simulink model "turbine"  (R2018b)
settings: Solver=ode1  StartTime=0.0  StopTime=100  FixedStep=0.1  RelTol=1e-3
PostLoadFcn:
  | , if any(exist('dsrtsu_mdlpostloadfcn', 'file') ~= 0), dsrtsu_mdlpostloadfcn('Execute', bdroot); end,
undefined symbols (not defined in the file): XXX
libraries: rtiethernetudplib x2
Description:
  | Standard RTI1401 template.
  | Supported MATLAB version:  R2018b.
settings Model: Tag=RTI1401  DSRTSU_INTERNAL_RTI_VER=530  DSRTSU_INTERNAL_RTI_TYPE=rti1401  RTICANMMDATA=struct('GeneralSetupData',struct('modelroot','C:\Users\akohlheb\working_files\OFF_RTS_PLC_API\dSpace','generalsettings',struct('filesettings',struct('destfolder',struct('Name','RTICANMM_FILES','Check',1),'buildfolder',struct('Name','.','Check',1),'AbsDestfolder',struct('Name','C:\Users\akohlheb\working_files\OFF_RTS_PLC_API\dSpace\RTICANMM_FILES'),'AbsBuildfolder',struct('Name','C:\Users\akohlheb\working_files\OFF_RTS_PLC_API\dSpace'))),'options',struct('addpaths',1,'rmpaths',1,'addtrcexclusion',logical(1),'cannavigator',struct('checkmonitoring',0),'show_usrtrc',0,'use_usrtrc',0),'advanced',struct('options',ones(1,100)),'MPSetup',{{}},'RTI',struct('Type','RTI1401','Ver','7.11','Date','02-Nov-2018'),'modelname','turbine','block','turbine'))  DSRTSU_INTERNAL_RTIFPGA=120  Creator=akohlheb  LastModifiedBy=akohlheb
settings OptimizationCC: BlockReduction=off  OptimizeBlockIOStorage=off  BufferReuse=off  GlobalBufferReuse=off  ExpressionFolding=off  LocalBlockOutputs=off  OptimizeDataStoreBuffers=off  BusAssignmentInplaceUpdate=off
settings DebuggingCC: LibraryContextMissingDiagnostic=none
settings HardwareCC: ProdBitPerPointer=32  ProdBitPerSizeT=32  ProdBitPerPtrDiffT=32  ProdLargestAtomicInteger=Integer  ProdEndianess=BigEndian  ProdWordSize=32  ProdHWDeviceType=Custom Processor->Custom  TargetIntDivRoundTo=Zero  TargetEndianess=BigEndian  TargetHWDeviceType=Custom Processor->Custom
settings SFSimCC: SimUseLocalCustomCode=off  MATLABDynamicMemAlloc=off
settings RTWCC: SystemTargetFile=rti1401.tlc  MakeCommand=make_rti  TemplateMakefile=rti1401.tmf  Description=dSPACE DS1401 Hardware Platform  RTWUseLocalCustomCode=off
settings CodeAppCC: StateflowObjectComments=on
settings STFCustomTargetCC: ParMdlRefBuildCompliant=on  SystemTargetFile=rti1401.tlc
settings GRTTargetCC: TargetLangStandard=C89/C90 (ANSI)  CompOptLevelCompliant=off  ConcurrentExecutionCompliant=off  CombineOutputUpdateFcns=off  MatFileLogging=off  CPPClassGenCompliant=off  UseToolchainInfoCompliant=off
settings ConfigComp: CovMetricSettings=dswe

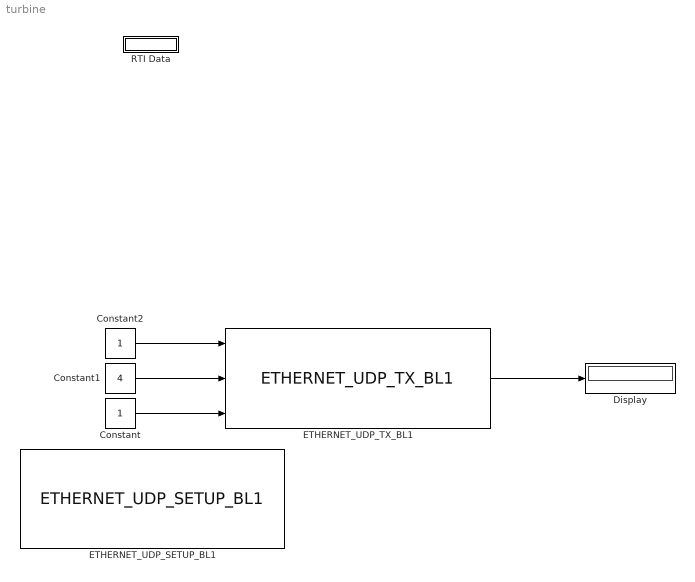
== system turbine ==
  Constant : Constant  OutDataTypeStr=boolean
  Constant1 : Constant  Value=4  OutDataTypeStr=int32
  Constant2 : Constant  OutDataTypeStr=uint32
  Display : Display
  ETHERNET_UDP_SETUP_BL1 : rtiethernetudplib/ETHERNET_UDP_SETUP_BL1  DSProperties=struct('RTI',struct('Version',uint32(1),'BlockType',struct('isSLSource',uint8(0),'isSLSink',uint8(0),'isHWSource',uint8(0),'isHWSink',uint8(0),'isSetup',uint8(0),'isInline',uint8(1),'isNonInline',uint8(1),'isInterrupt',uint8(0),'isChannelwise',uint8(0)),'IOBoardType','DSETHERNETUDP','UnitType','ETHUDP','Identifier','SETUP','DialogType','ML','BlockSet','RTIETHERNETUDP','SlaveProcessor','NONE'))  RTIBlockInterface=struct('OutputPortsActive',0,'OutputPortsWidth',int32(1),'DialogFcn','rtiethernetudpsetupgui','InitLevel',3,'BlockDisplay',{{['Ethernet UDP Setup\nInterface Name: rti_ethernet_interface_name\nBoard Type: ETH Type 1\nModule: 1\nLocal IP Address: XXX.XXX.XXX.XXX'],'center'}},'IconTransparency','on','BlockName',struct('Token',{{'ETHERNET_UDP_SETUP_BL1'}}))  RTIBlockParameters=struct('BoardType',{{1,'OFF',[]}},'ModuleNo',{{1,'ON',[1 16]}},'ChannelNo',{{1,'ON',[1 2]}},'InterfaceName',{{'rti_ethernet_interface_name','OFF',[]}},'LocalIpAddress',{{'XXX.XXX.XXX.XXX','OFF',[]}},'EnableSocket1',{{0,'OFF',[0 1]}},'LocalPortSocket1',{{5000,'OFF',[0 65535]}},'RemoteIpAddrSocket1',{{'XXX.XXX.XXX.XXX','OFF',[]}},'RemotePortSocket1',{{5000,'OFF',[0 65535]}},'EnableSocket2',{{0,'OFF',[0 1]}},'LocalPortSocket2',{{5001,'OFF',[0 65535]}},'RemoteIpAddrSocket2',{{'XXX.XXX.XXX.XXX','OFF',[]}},'RemotePortSocket2',{{5001,'OFF',[0 65535]}},'EnableSocket3',{{0,'OFF',[0 1]}},'LocalPortSocket3',{{5002,'OFF',[0 65535]}},'RemoteIpAddrSocket3',{{'XXX.XXX.XXX.XXX','OFF',[]}},'RemotePortSocket3',{{5002,'OFF',[0 65535]}},'EnableSocket4',{{0,'OFF',[0 1]}},'LocalPortSocket4',{{5003,'OFF',[0 65535]}},'RemoteIpAddrSocket4',{{'XXX.XXX.XXX.XXX','OFF',[]}},'RemotePortSocket4',{{5003,'OFF',[0 65535]}},'LocalIpAddrHex',{{0,'OFF',[]}},'RemoteIpAddrSocket1Hex',{{0,'OFF',[]}},'RemoteIpAddrSocket2Hex',{{0,'OFF',[]}},'RemoteIpAddrSocket3Hex',{{0,'OFF',[]}},'RemoteIpAddrSocket4Hex',{{0,'OFF',[]}})  RTISFcnParameters=struct('BoardType','double','ModuleNo','double','ChannelNo','double','InterfaceName','char','LocalIpAddress','char','EnableSocket1','double','LocalPortSocket1','double','RemoteIpAddrSocket1','char','RemotePortSocket1','double','EnableSocket2','double','LocalPortSocket2','double','RemoteIpAddrSocket2','char','RemotePortSocket2','double','EnableSocket3','double','LocalPortSocket3','double','RemoteIpAddrSocket3','char','RemotePortSocket3','double','EnableSocket4','double','LocalPortSocket4','double','RemoteIpAddrSocket4','char','RemotePortSocket4','double','LocalIpAddrHex','double','RemoteIpAddrSocket1Hex','double','RemoteIpAddrSocket2Hex','double','RemoteIpAddrSocket3Hex','double','RemoteIpAddrSocket4Hex','double')  RTIBlockParaDefault=struct('BoardType',1,'ModuleNo',1,'ChannelNo',1,'InterfaceName','rti_ethernet_interface_name','LocalIpAddress','XXX.XXX.XXX.XXX','EnableSocket1',0,'LocalPortSocket1',5000,'RemoteIpAddrSocket1','XXX.XXX.XXX.XXX','RemotePortSocket1',5000,'EnableSocket2',0,'LocalPortSocket2',5001,'RemoteIpAddrSocket2','XXX.XXX.XXX.XXX','RemotePortSocket2',5001,'EnableSocket3',0,'LocalPortSocket3',5002,'RemoteIpAddrSocket3','XXX.XXX.XXX.XXX','RemotePortSocket3',5002,'EnableSocket4',0,'LocalPortSocket4',5003,'RemoteIpAddrSocket4','XXX.XXX.XXX.XXX','RemotePortSocket4',5003,'LocalIpAddrHex',0,'RemoteIpAddrSocket1Hex',0,'RemoteIpAddrSocket2Hex',0,'RemoteIpAddrSocket3Hex',0,'RemoteIpAddrSocket4Hex',0)
      settings: SourceProductName=dSPACE RTI Ethernet (UDP) Blockset
  ETHERNET_UDP_TX_BL1 : rtiethernetudplib/ETHERNET_UDP_TX_BL1  InterfaceName=rti_ethernet_interface_name  BoardType=ETH Type 1  ModuleNo=1  ChannelNo=1  SocketNo=1  MaxMessageSize=4  SendTimeout=0.0005  LocalSocket=XXX.XXX.XXX.XXX:5000  RemoteSocket=XXX.XXX.XXX.XXX:5000  DSProperties=struct('RTI',struct('Version',uint32(2),'BlockType',struct('isSLSource',uint8(1),'isSLSink',uint8(1),'isHWSource',uint8(1),'isHWSink',uint8(1),'isSetup',uint8(0),'isInline',uint8(1),'isNonInline',uint8(1),'isInterrupt',uint8(0),'isChannelwise',uint8(1)),'IOBoardType','DSETHERNETUDP','UnitType','ETHUDP','Identifier','TX','DialogType','SL','BlockSet','RTIETHERNETUDP','SlaveProcessor','NONE'))  RTIBlockInterface=struct('OutputPortsWidth',int32(1),'OutputPortsActive',1,'OutputPortsName',{{'Status'}},'OutputPortsDataType',{{'SS_UINT16'}},'InputPortsWidth',int32([1 1 1]),'InputPortsActive',[1 1 1],'InputPortsName',{{'Data',['Message Size'],'Enable'}},'InputPortsDataType',{{'SS_UINT32','SS_INT32','SS_BOOLEAN'}},'BlockDisplay',{{['Ethernet UDP Transmit\nBoard Type: ETH Type 1\nModule: 1\nSocket: 1\nMaximum Message Size: 4'],'center'}},'IconTransparency','on','InitLevel',3,'BlockName',struct('Token',{{'ETHERNET_UDP_TX_BL1'}}),'MaskDescription',['To send messages via the Ethernet UDP interface.'])  RTIBlockParameters=struct('InterfaceName',{{'rti_ethernet_interface_name','OFF',[]}},'BoardType',{{1,'OFF',[]}},'ModuleNo',{{1,'OFF',[1 16]}},'ChannelNo',{{1,'OFF',[1 2]}},'SocketNo',{{1,'OFF',[1 4]}},'MaxMessageSize',{{4,'ON',[1 1472]}},'SendTimeout',{{0.0005,'ON',[1e-5 2]}},'LocalSocket',{{'XXX.XXX.XXX.XXX:5000','OFF',[]}},'RemoteSocket',{{'XXX.XXX.XXX.XXX:5000','OFF',[]}})  RTISFcnParameters=struct('InterfaceName','char','BoardType','double','ModuleNo','double','ChannelNo','double','SocketNo','double','MaxMessageSize','double','SendTimeout','double','LocalSocket','char','RemoteSocket','char')  RTIBlockParaDefault=struct('InterfaceName','rti_ethernet_interface_name','BoardType',1,'ModuleNo',1,'ChannelNo',1,'SocketNo',1,'MaxMessageSize',625,'SendTimeout',0.0005,'LocalSocket','XXX.XXX.XXX.XXX:5000','RemoteSocket','XXX.XXX.XXX.XXX:5000')
      settings: SourceProductName=dSPACE RTI Ethernet (UDP) Blockset
  RTI Data : Subsystem  Tag=struct('RTIDataServer',struct('RTIDataServerVs','2','RTIModelDescription','struct(''main'',''turbine'',''sub'','''',''isMp'',0)'))  LoadFcn="if exist('rtidc'), try,  rtidc('DataHostBlockClbLoad', gcbh); catch, disp(['Warning: ''LoadFcn'' for RTI Data block failed: ' lasterr]); end, end,"  mask(RTI_DATA_HOST){}
      mask help:
      | RTI Data Block.
      | This block is used by RTI to store internal model-dependent data.
      | Please keep this block on the root level of the model. Deleting this block will result in data loss.
      |
      | NEVER DELETE OR COPY THIS BLOCK!
      settings: CopyFcn="if exist('rtidc'), try,  rtidc('DataHostBlockClbCopy', gcbh); catch, disp(['Warning: ''CopyFcn'' for RTI Data block failed: ' lasterr]); end, end,"  DeleteFcn="if exist('rtidc'), try,  rtidc('DataHostBlockClbDelete', gcbh); catch, disp(['Warning: ''DeleteFcn'' for RTI Data block failed: ' lasterr]); end, end,"  ModelCloseFcn="if exist('rtidc'), try,  rtidc('DataHostBlockClbModelClose', gcbh); catch, disp(['Warning: ''ModelCloseFcn'' for RTI Data block failed: ' lasterr]); end, end,"  PreSaveFcn="if exist('rtidc'), try,  rtidc('DataHostBlockClbPreSave', gcbh); catch, disp(['Warning: ''PreSaveFcn'' for RTI Data block failed: ' lasterr]); end, end,"  PostSaveFcn="if exist('rtidc'), try,  rtidc('DataHostBlockClbPostSave', gcbh); catch, disp(['Warning: ''PostSaveFcn'' for RTI Data block failed: ' lasterr]); end, end,"  NameChangeFcn="if exist('rtidc'), try,  rtidc('DataHostBlockClbNameChange', gcbh); catch, disp(['Warning: ''NameChangeFcn'' for RTI Data block failed: ' lasterr]); end, end,"
      mask Help:
      | RTI Data Block.
      | This block is used by RTI to store internal model-dependent data.
      | Please keep this block on the root level of the model. Deleting this block will result in data loss.
      | 
      | NEVER DELETE OR COPY THIS BLOCK!
      mask Display:
      | text(0.5, 0.5, 'RTI Data', 'HorizontalAlignment', 'center');
      | plot([1 0]);
  wires:
  Constant/1 -> ETHERNET_UDP_TX_BL1/3
  Constant1/1 -> ETHERNET_UDP_TX_BL1/2
  ETHERNET_UDP_TX_BL1/1 -> Display/1
  Constant2/1 -> ETHERNET_UDP_TX_BL1/1

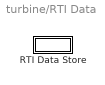
== system turbine/RTI Data ==
  RTI Data Store : Subsystem  Tag="struct('private',struct('version',struct('dsVer',uint32(2),'dsVerCreation',uint32(2),'RTI',struct('ver','7.11','type','RTI1401')),'access',struct('type','Model','isPerm',1,'created',['13-Jan-2026 13:51:52'],'modified',['14-Jan-2026 18:15:54'],'location','')),'public',struct('main',struct('data',[]),'sub',struct('name',{{'turbine'}},'data',{{struct('TH',struct('thTaskInfo',struct('taskType',{'TIMER','HWINT','TMRINT','SWINT','GLINT'},'tasksNumOf',{1,0,0,0,0},'srcIds',{{'TIMERA'},{},{},{},{}},'taskNames',{{['Timer Task 1']},{},{},{},{}})),'th_tc',struct('dataType','TASK','taskGroupId','','taskGroupList',{{}},'taskSchedulingPolicy','FCFS','taskType','TIMER','blkh',-1,'srcId','TIMERA','srcSgnName',['Timer A interrupt'],'srcCpuName','','taskName',['Timer Task 1  [0.001] s'],'taskNameDisplayExt','','smplTime',0.001,'smplTimeOffs',0,'hasFixedPriority',0,'priority',1,'hasFixedOvc',0,'ovcType',1,'ovcMax',1),'tc_th',struct('dataType','TASK','taskGroupId','','taskGroupList',{{}},'taskSchedulingPolicy','FCFS','taskType','TIMER','blkh',-1,'srcId','TIMERA','srcSgnName',['Timer A interrupt'],'srcCpuName','','taskName',['Timer Task 1  [0.001] s'],'taskNameDisplayExt','','smplTime',0.001,'smplTimeOffs',0,'hasFixedPriority',0,'priority',1,'hasFixedOvc',0,'ovcType',1,'ovcMax',1))}})))"  mask(RTI_DATA_STORE){}
      mask help:
      | RTI Data Store Block. This block is used by RTI to store internal model dependent data. Deleting this block will result in data loss.
      |
      | NEVER DELETE, COPY, OR MODIFY THIS BLOCK!
      mask Help:
      | RTI Data Store Block. This block is used by RTI to store internal model dependent data. Deleting this block will result in data loss.
      | 
      | NEVER DELETE, COPY, OR MODIFY THIS BLOCK!
      mask Display: text(0.5, 0.5, ' ', 'HorizontalAlignment', 'center');

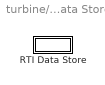
== system turbine/RTI Data/RTI Data Store ==
  RTI Data Store : Subsystem  mask(RTI_DATA_STORE){}
      mask help:
      | RTI Data Store Block. This block is used by RTI to store internal model dependent data. Deleting this block will result in data loss.
      |
      | NEVER DELETE, COPY, OR MODIFY THIS BLOCK!
      mask Help:
      | RTI Data Store Block. This block is used by RTI to store internal model dependent data. Deleting this block will result in data loss.
      | 
      | NEVER DELETE, COPY, OR MODIFY THIS BLOCK!
      mask Display: text(0.5, 0.5, ' ', 'HorizontalAlignment', 'center');

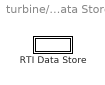
== system turbine/RTI Data/RTI Data Store/RTI Data Store ==
  RTI Data Store : Subsystem  mask(RTI_DATA_STORE){}
      mask help:
      | RTI Data Store Block. This block is used by RTI to store internal model dependent data. Deleting this block will result in data loss.
      |
      | NEVER DELETE, COPY, OR MODIFY THIS BLOCK!
      mask Help:
      | RTI Data Store Block. This block is used by RTI to store internal model dependent data. Deleting this block will result in data loss.
      | 
      | NEVER DELETE, COPY, OR MODIFY THIS BLOCK!
      mask Display: text(0.5, 0.5, ' ', 'HorizontalAlignment', 'center');

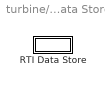
== system turbine/RTI Data/RTI Data Store/RTI Data Store/RTI Data Store ==
  RTI Data Store : Subsystem  mask(RTI_DATA_STORE){}
      mask help:
      | RTI Data Store Block. This block is used by RTI to store internal model dependent data. Deleting this block will result in data loss.
      |
      | NEVER DELETE, COPY, OR MODIFY THIS BLOCK!
      mask Help:
      | RTI Data Store Block. This block is used by RTI to store internal model dependent data. Deleting this block will result in data loss.
      | 
      | NEVER DELETE, COPY, OR MODIFY THIS BLOCK!
      mask Display: text(0.5, 0.5, ' ', 'HorizontalAlignment', 'center');

== system turbine/RTI Data/RTI Data Store/RTI Data Store/RTI Data Store/RTI Data Store ==
